simulink model "PID_Model_28May2025"  (R2024b)
settings: Solver=FixedStepAuto  StartTime=0.0  StopTime=80  RelTol=1e-3
undefined symbols (not defined in the file or in its folder): DiscIntNeverNeededParam, gaussian
libraries: SignalEditorBlockLib x2, simulink x2, sdolib x1, slpidlib x1
settings Model: Creator=shak2  LastModifiedBy=shak2
settings DataIOCC: SaveOutput=off  SignalLogging=off  SaveTime=off

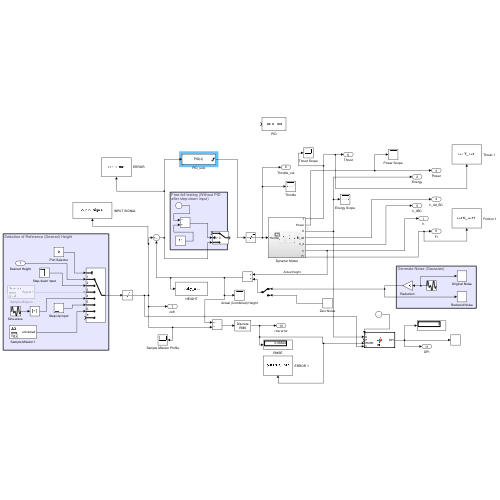
[thumbnail: Simulink's stored preview of the top-level diagram]
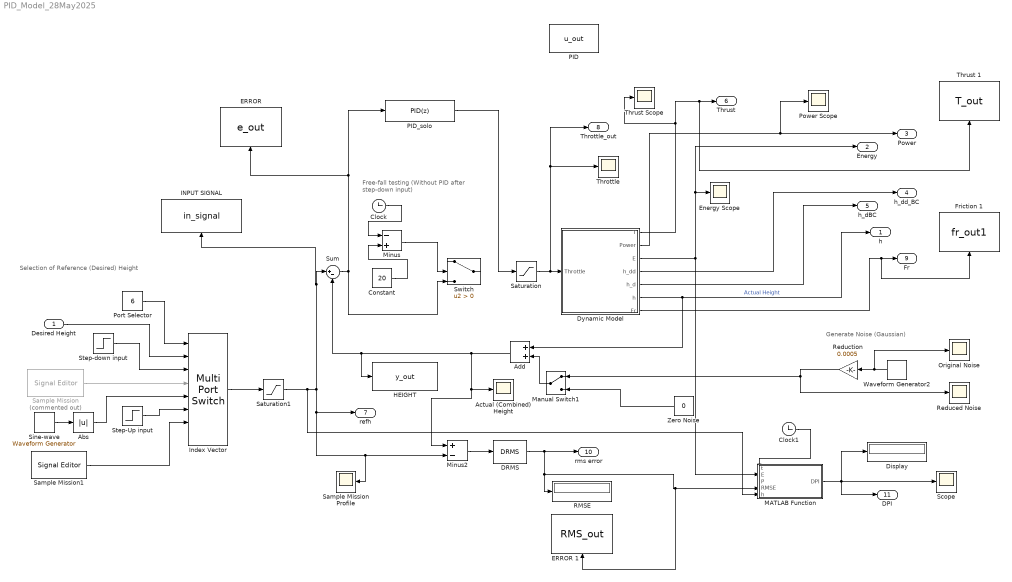
== system PID_Model_28May2025 ==
  note: Selection of Reference (Desired) Height
  note: Free-fall testing (Without PID
      | after step-down input)
  note: Generate Noise (Gaussian)
  Desired Height : Inport
  Abs : Abs  SaturateOnIntegerOverflow=off
  Actual (Combined) Height : Scope
  Add : Sum
  Clock : Clock
  Clock1 : Clock
  Constant : Constant  Value=20
  DRMS : sdolib/RMS Blocks/DRMS  Ts=0.05
  Display : Display
  Dynamic Model : Subsystem
  "ERROR " : ToWorkspace  VariableName=e_out  SaveFormat=Structure With Time  SampleTime=0.05
      settings: Save2DSignal=2-D array (concatenate along first dimension)
  ERROR 1 : ToWorkspace  VariableName=RMS_out  SaveFormat=Structure With Time  SampleTime=0.05
      settings: Save2DSignal=2-D array (concatenate along first dimension)
  Energy Scope : Scope
  Friction 1 : ToWorkspace  VariableName=fr_out1  SaveFormat=Structure With Time  SampleTime=0.05
      settings: Save2DSignal=2-D array (concatenate along first dimension)
  HEIGHT : ToWorkspace  VariableName=y_out  SaveFormat=Structure With Time  SampleTime=0.05
      settings: Save2DSignal=2-D array (concatenate along first dimension)
  INPUT SIGNAL : ToWorkspace  VariableName=in_signal  SaveFormat=Structure With Time  SampleTime=0.05
      settings: Save2DSignal=2-D array (concatenate along first dimension)
  Index Vector : MultiPortSwitch  Inputs=6  DataPortForDefault=Additional data port  DiagnosticForDefault=None  SaturateOnIntegerOverflow=off  InputSameDT=off
  MATLAB Function : MATLAB Function  TreatAsAtomicUnit=on
  Manual Switch1 : ManualSwitch
  Minus : Sum  Inputs=-+
  Minus2 : Sum  Inputs=+-
  Original Noise : Scope
  PID : ToWorkspace  VariableName=u_out  SaveFormat=Structure With Time  SampleTime=0.05
      settings: Save2DSignal=2-D array (concatenate along first dimension)
  PID_solo : slpidlib/PID Controller  Controller=PID  Form=Parallel  TimeDomain=Discrete-time  UseExternalTs=off  SampleTime=-1  IntegratorMethod=Forward Euler  FilterMethod=Forward Euler  ControllerParametersSource=internal  P=106.9  I=71.8  UseKiTs=off  D=38.6  UseExternalDerivativeSource=off  N=14  UseFilter=on  TunerSelectOption=Transfer Function Based (PID Tuner App)  InitialConditionSource=internal  InitialConditionForIntegrator=0  InitialConditionForFilter=0  DifferentiatorICPrevScaledInput=0  ExternalReset=none  TrackingMode=off  Kt=1  LimitOutput=on  SatLimitsSource=internal  UpperSaturationLimit=inf  LowerSaturationLimit=-inf  LinearizeAsGain=off  AntiWindupMode=clamping  Kb=1  LimitIntegrator=off  UpperIntegratorSaturationLimit=inf  LowerIntegratorSaturationLimit=-inf  POutMin=[]  POutMax=[]  IOutMin=[]  IOutMax=[]  DOutMin=[]  DOutMax=[]  NOutMin=[]  NOutMax=[]  SumOutMin=[]  SumOutMax=[]  SaturationOutMin=[]  SaturationOutMax=[]  PParamMin=[]  PParamMax=[]  IParamMin=[]  IParamMax=[]  DParamMin=[]  DParamMax=[]  NParamMin=[]  NParamMax=[]  KbParamMin=[]  KbParamMax=[]  KtParamMin=[]  KtParamMax=[]  KbOutMin=[]  KbOutMax=[]  KtOutMin=[]  KtOutMax=[]  IntegratorOutMin=[]  IntegratorOutMax=[]  FilterOutMin=[]  FilterOutMax=[]  SumI1OutMin=[]  SumI1OutMax=[]  SumI2OutMin=[]  SumI2OutMax=[]  SumI3OutMin=[]  SumI3OutMax=[]  SumI4OutMin=[]  SumI4OutMax=[]  SumDOutMin=[]  SumDOutMax=[]  DifferentiatorOutMin=[]  DifferentiatorOutMax=[]  FilterDiffOutCoefMin=[]  FilterDiffOutCoefMax=[]  ReciprocalOutMin=[]  ReciprocalOutMax=[]  SumDenOutMin=[]  SumDenOutMax=[]  SumNumOutMin=[]  SumNumOutMax=[]  DivideOutMin=[]  DivideOutMax=[]  UdiffTsProdOutMin=[]  UdiffTsProdOutMax=[]  NTsProdOutMin=[]  NTsProdOutMax=[]  UintegralTsProdOutMin=[]  UintegralTsProdOutMax=[]  UngainTsProdOutMin=[]  UngainTsProdOutMax=[]  ClampingZeroOutDataTypeStr=Inherit: Inherit via back propagation  ClampingZeroOutMin=[]  ClampingZeroOutMax=[]  FilterDenConstantOutDataTypeStr=Inherit: Inherit via back propagation  FilterDenConstantOutMin=[]  FilterDenConstantOutMax=[]  PCopyOutDataTypeStr=Inherit: Inherit via back propagation  PCopyOutMin=[]  PCopyOutMax=[]  NCopyOutDataTypeStr=Inherit: Inherit via back propagation  NCopyOutMin=[]  NCopyOutMax=[]  IntegratorContinuousStateAttributes=''  IntegratorStateMustResolveToSignalObject=off  IntegratorRTWStateStorageClass=Auto  FilterContinuousStateAttributes=''  FilterStateMustResolveToSignalObject=off  FilterRTWStateStorageClass=Auto  ParallelPVariant=InternalParameters  IdealPVariant=Disabled  IVariant=InternalParameters  DVariant=InternalParameters  IntegratorVariant=Discrete  SatVariant=Enabled  AWVariant=DiscClampingParallel  PCopyVariant=Disabled  TRVariant=Disabled  FdbkBlocksVariant=Forward  IdealPFdbkVariant=Disabled  SatFdbkVariant=Disabled  DerivativeFilterVariant=ForwardEulerFilter  NVariant=InternalParameters  NCopyVariant=Disabled  FilterICVariant=InternalICsFilter  IntegratorICVariant=InternalICs  ExternalResetVariant=Disabled  TRSumVariant=Passthrough  SumFdbkVariant=Disabled  SumVariant=Sum_PID  TsampFilterVariant=InternalTs  TsampNgainVariant=Passthrough  TsampIntegralVariant=Disabled_SignalSpec  ExternalSaturationOutDataTypeStr=Inherit: Same as second input  DerivativeSourceVariant=ErrorSignal  PreIntVariant=InternalPreInt
      settings: LibrarySourceBlock=simulink/Discrete/Discrete PID Controller
  Port Selector : Constant  Value=6
  Power Scope : Scope
  RMSE : Display
  Reduced Noise : Scope
  Reduction : Gain  Gain=0.0005
  Sample Mission : SignalEditorBlockLib/Signal Editor  Commented=on  FileName=samplemission.mat  ActiveScenario=Scenario  ActiveSignal=Signal 1  IsBus=off  OutputBusObjectStr=Bus: BusObject  SampleTime=0.05  ZeroCross=off  OutputAfterFinalValue=Setting to zero  Unit=inherit  PreserveSignalName=on  ApplySigPropsToAllScenarios=on  ApplySigPropsToAllSignals=off
  Sample Mission Profile : Scope
  Sample Mission1 : SignalEditorBlockLib/Signal Editor  FileName=ds2 1.mat  ActiveScenario=ds2  ActiveSignal=unnamed  IsBus=off  OutputBusObjectStr=Bus: BusObject  SampleTime=0  ZeroCross=off  OutputAfterFinalValue=Setting to zero  Unit=inherit  PreserveSignalName=on  ApplySigPropsToAllScenarios=on  ApplySigPropsToAllSignals=off
  Saturation : Saturate  UpperLimit=90  LowerLimit=0
  Saturation1 : Saturate  UpperLimit=1.44  LowerLimit=0
  Scope : Scope
  "Sine-wave " : simulink/Sources/Waveform Generator  OutMin=[]  OutMax=[]  OutDataTypeStr=double  SelectedSignal=1  Signals=sin('Amplitude', 0.2, 'Frequency', 0.1, 'Phase', 0)  BlockNames=MultiportSwitch_e159a769fb8743c  SampleTime=0.05
  Step-Up input : Step  Time=10  SampleTime=0.05
  Step-down input : Step  Time=20  Before=1.44  After=0  SampleTime=0.05
  Sum : Sum  Inputs=|+-
  Switch : Switch  Criteria=u2 > Threshold  SaturateOnIntegerOverflow=off  InputSameDT=off
  Throttle : Scope
  Thrust 1 : ToWorkspace  VariableName=T_out  SaveFormat=Structure With Time  SampleTime=0.05
      settings: Save2DSignal=2-D array (concatenate along first dimension)
  Thrust Scope : Scope
  Waveform Generator2 : simulink/Sources/Waveform Generator  OutMin=[]  OutMax=[]  OutDataTypeStr=double  SelectedSignal=1  Signals=gaussian('Mean',0,'Variance',10,'Seed',1)  BlockNames=MultiportSwitch_20caeb741fc64b7  SampleTime=0.05
  Zero Noise : Constant  Value=0  OutDataTypeStr=Inherit: Inherit via back propagation
  h : Outport
  Energy : Outport  Port=2
  Power : Outport  Port=3
  h_dd_BC : Outport  Port=4
  h_dBC : Outport  Port=5
  Thrust : Outport  Port=6
  refh : Outport  Port=7
  Throttle_out : Outport  Port=8
  Fr : Outport  Port=9
  rms error : Outport  Port=10
  DPI : Outport  Port=11
  wires:
  Dynamic Model/1(T) -> Thrust 1/1, Thrust/1, Thrust Scope/1
  Dynamic Model/2(Power) -> Power Scope/1, Power/1
  Dynamic Model/3(E) -> Energy/1, Energy Scope/1, MATLAB Function/2(E)
  Dynamic Model/4(h_dd) -> h_dd_BC/1
  Dynamic Model/5(h_d) -> h_dBC/1
  Dynamic Model/6(h) -> Add/1, h/1  "Actual Height"
  Saturation/1 -> Throttle_out/1, Throttle/1, Dynamic Model/1(Throttle)
  Desired Height/1 -> Index Vector/2
  Waveform Generator2/1 -> Original Noise/1, Reduction/1
  Manual Switch1/1 -> Add/2
  Zero Noise/1 -> Manual Switch1/2
  Sum/1 -> PID_solo/1, "ERROR "/1, Switch/3
  Minus/1 -> Switch/2
  Clock/1 -> Minus/1
  Constant/1 -> Minus/2
  Sample Mission/1 -> Index Vector/4
  Step-down input/1 -> Index Vector/3
  Port Selector/1 -> Index Vector/1
  Abs/1 -> Index Vector/5
  "Sine-wave "/1 -> Abs/1
  Reduction/1 -> Reduced Noise/1, Manual Switch1/1
  Index Vector/1 -> Saturation1/1
  Dynamic Model/7(Fr) -> Friction 1/1, Fr/1
  Add/1 -> HEIGHT/1, Sum/2, Minus2/1, Actual (Combined) Height/1
  Step-Up input/1 -> Index Vector/6
  Sample Mission1/1 -> Index Vector/7
  Minus2/1 -> DRMS/1
  DRMS/1 -> ERROR 1/1, MATLAB Function/4(RMSE), RMSE/1, rms error/1
  MATLAB Function/1(DPI) -> Scope/1, Display/1, DPI/1
  Clock1/1 -> MATLAB Function/1(t)
  Saturation1/1 -> MATLAB Function/5(h), Minus2/2, Sample Mission Profile/1, refh/1, INPUT SIGNAL/1, Sum/1
  PID_solo/1 -> Saturation/1

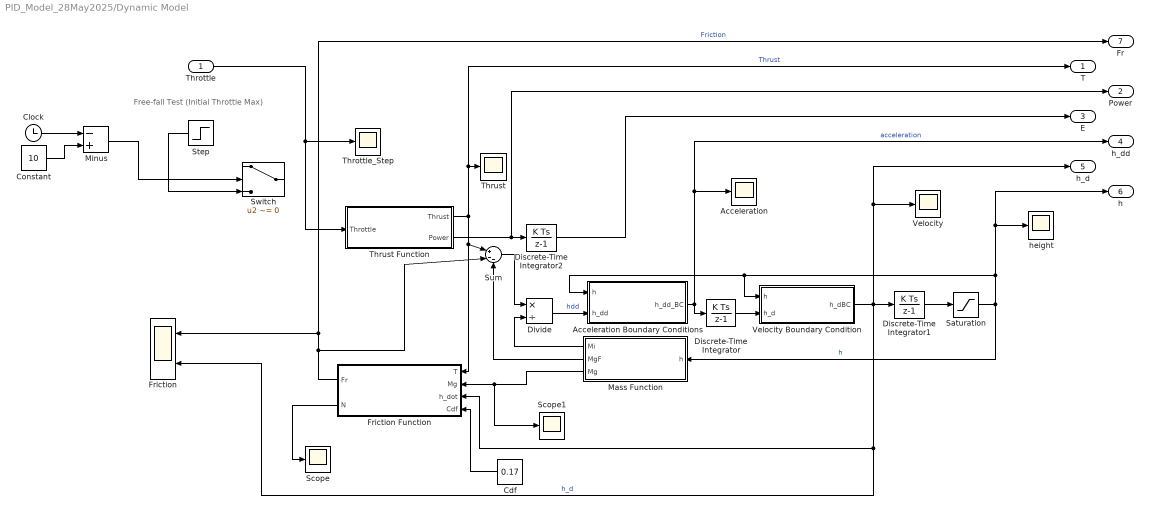
== system PID_Model_28May2025/Dynamic Model ==
  note: Free-fall Test (Initial Throttle Max)
  Throttle : Inport
  Acceleration : Scope
  Acceleration Boundary Conditions : MATLAB Function  TreatAsAtomicUnit=on
  Cdf : Constant  Value=0.17
  Clock : Clock
  Constant : Constant  Value=10
  Discrete-Time Integrator : DiscreteIntegrator  SampleTime=-1  ICPrevOutput=DiscIntNeverNeededParam  ICPrevScaledInput=DiscIntNeverNeededParam
  Discrete-Time Integrator1 : DiscreteIntegrator  SampleTime=-1  ICPrevOutput=DiscIntNeverNeededParam  ICPrevScaledInput=DiscIntNeverNeededParam
  Discrete-Time Integrator2 : DiscreteIntegrator  SampleTime=-1  ICPrevOutput=DiscIntNeverNeededParam  ICPrevScaledInput=DiscIntNeverNeededParam
  Divide : Product  Inputs=*/
  Friction : Scope  NumInputPorts=2
  Friction Function : MATLAB Function  TreatAsAtomicUnit=on
  Mass Function : MATLAB Function  TreatAsAtomicUnit=on
  Minus : Sum  Inputs=-+
  Saturation : Saturate  UpperLimit=1.44  LowerLimit=0
  Scope : Scope
  Scope1 : Scope
  Step : Step  Time=10  Before=1  After=0  SampleTime=0
  Sum : Sum  Inputs=|+--
  Switch : Switch  Criteria=u2 ~= 0  SaturateOnIntegerOverflow=off  InputSameDT=off
  Throttle_Step : Scope
  Thrust : Scope
  Thrust Function : MATLAB Function  TreatAsAtomicUnit=on
  Velocity : Scope
  Velocity Boundary Condition : MATLAB Function  TreatAsAtomicUnit=on
  height : Scope
  T : Outport
  Power : Outport  Port=2
  E : Outport  Port=3
  h_dd : Outport  Port=4
  h_d : Outport  Port=5
  h : Outport  Port=6
  Fr : Outport  Port=7
  wires:
  Divide/1 -> Acceleration Boundary Conditions/2(h_dd)  "hdd"
  Saturation/1 -> Velocity Boundary Condition/1(h), Acceleration Boundary Conditions/1(h), h/1, height/1, Mass Function/1(h)  "h"
  Thrust Function/2(Power) -> Power/1, Discrete-Time Integrator2/1
  Sum/1 -> Divide/1
  Mass Function/1(Mi) -> Divide/2
  Discrete-Time Integrator2/1 -> E/1
  Thrust Function/1(Thrust) -> T/1, Thrust/1, Friction Function/1(T), Sum/1  "Thrust"
  Acceleration Boundary Conditions/1(h_dd_BC) -> Discrete-Time Integrator/1, h_dd/1, Acceleration/1  "acceleration"
  Discrete-Time Integrator/1 -> Velocity Boundary Condition/2(h_d)
  Mass Function/2(MgF) -> Sum/3
  Discrete-Time Integrator1/1 -> Saturation/1
  Friction Function/1(Fr) -> Fr/1, Friction/1, Sum/2  "Friction"
  Velocity Boundary Condition/1(h_dBC) -> Friction/2, Friction Function/3(h_dot), Velocity/1, h_d/1, Discrete-Time Integrator1/1  "h_d"
  Step/1 -> Switch/3
  Constant/1 -> Minus/2
  Clock/1 -> Minus/1
  Minus/1 -> Switch/2
  Cdf/1 -> Friction Function/4(Cdf)
  Friction Function/2(N) -> Scope/1
  Throttle/1 -> Throttle_Step/1, Thrust Function/1(Throttle)
  Mass Function/3(Mg) -> Scope1/1, Friction Function/2(Mg)

== matlab function PID_Model_28May2025/Dynamic Model/Mass Function ==
  data: Mi output; MgF output; h input; Mg output
function [Mi, MgF, Mg] = MassFunction(h)
%Given Masses in Kg

Mm = 0.328; % 2 x (Motor Mass + ESC + Propellor)
Ma = 0.05; % Total Arm Mass
Mk = 0.15; % Given Cart Mass

M_constant = Mk + Mm + Ma;

Mc = 2*(0.095*h + 0.0532); %mass of cable is function of height

Mg = M_constant + Mc; %gravitational load
Mi= Mg + 0.8;% gravitational + carriage + counterweight + 8 sliders

MgF = Mg * 9.81;

== matlab function PID_Model_28May2025/Dynamic Model/Thrust Function ==
  data: Throttle input; Thrust output; Power output
function [Thrust, Power]= ThrustFunction(Throttle)

S_t = Throttle/100;

%Throttle to Thrust

% Polyfit 6th Order

a = 0.451880436962741;
b = -1.486027191210204;
c = 1.797219095509746;
d = -0.984318732289241;
e = 0.241341383767270;
f = -0.007579836329288;

Thrust = 2 * (1.0e+03) * (a*S_t^6 + b*S_t^5 + c*S_t^4 + d*S_t^3 + e*S_t^2 + f*S_t ); 

% Polyfit 6th Order

a = 1.401054302991919;
b = -4.543527223865324;
c = 5.384918481145972;
d = -2.871958912880594;
e = 0.697342980048495;
f = -0.033090224044331;

Power = 2 * (1.0e+04) * (a*S_t^6 + b*S_t^5 + c*S_t^4 + d*S_t^3 + e*S_t^2 + f*S_t);

== matlab function PID_Model_28May2025/Dynamic Model/Friction Function ==
  data: T input; Mg input; h_dot input; Cdf input; Fr output; N output
function [Fr,N] = FrictionFunction(T, Mg, h_dot, Cdf)

%% geometry *CURRENTLY PLACEHOLDER VALUES*
l_t = 0.01; %Thrust Moment Arm
l_cg = 0.013922; %Centre of Gravity Moment Arm
l_c = 0.2104; %Length of carriage Moment

FrStatic = 0.26 * 9.81; %Static Friction

N = abs((T*l_t - Mg*9.81*l_cg)/l_c); %Normal reaction force 
    
if abs(h_dot) == 0
        Fr = FrStatic; %static friction
else
    Fr = sign(h_dot) * Cdf*N;
end

== matlab function PID_Model_28May2025/Dynamic Model/Acceleration Boundary Conditions ==
  data: h input; h_dd input; h_dd_BC output
function h_dd_BC = Accel_BC(h,h_dd)
% Acceleration must be 0 at the top and bottom
if (h <= 0 && h_dd < 0) || (h >= 1.44 && h_dd > 0)
    h_dd_BC = 0;
else
    h_dd_BC = h_dd;
end

== matlab function PID_Model_28May2025/Dynamic Model/Velocity Boundary Condition ==
  data: h input; h_d input; h_dBC output
function h_dBC = Vel_BC(h, h_d)

if (h==0 && h_d < 0) || (h==1.44 && h_d > 0)
    h_dBC = 0;
else
    h_dBC = h_d;
end

== matlab function PID_Model_28May2025/MATLAB Function ==
  data: t input; DPI output; E input; P input; RMSE input; h input
function DPI = fcn(t, E, P, RMSE, h)
DPI = 70 * (0.3 * E / (2 * P * t) + 0.4 * (RMSE/h))^(-1);
